simulink model "simumdl"  (Simulink 7.6)
settings: Solver=ode45  StartTime=0.0  StopTime=Tend  RelTol=1e-3
values from neighbouring files (symbols this model uses):
  A = 1    [contsid_MISO.m]
  B = [10 30]    [contsid_Hammerstein1.m]    (also in contsid_MISO.m = cell(1,2); B{1} = B1; B{2} = B2; contsid_RIVC.m = [2]; contsid_tutorial4.m = [-6400 1600]; contsid_tutorial5.m = K*wn^2*num)
  C = [1]    [contsid_Hammerstein1.m]    (also in contsid_HammersteinWiener1.m = sys0_ss.C; contsid_RIVC.m = [1 0.9])
  D = [1]    [contsid_Hammerstein1.m]    (also in contsid_HammersteinWiener1.m = sys0_ss.D; contsid_RIVC.m = [1 -1 .2])
  Dc = [1 0]    [contsid_closedloop1.m]
undefined symbols (not defined in the file or in its folder): Ac, Bc, Cc, Tsd
settings Model: Creator=pakjit  LastModifiedBy=pakjit
settings DataIOCC: LimitDataPoints=off  TimeSaveName=toutsim  OutputSaveName=youtsim

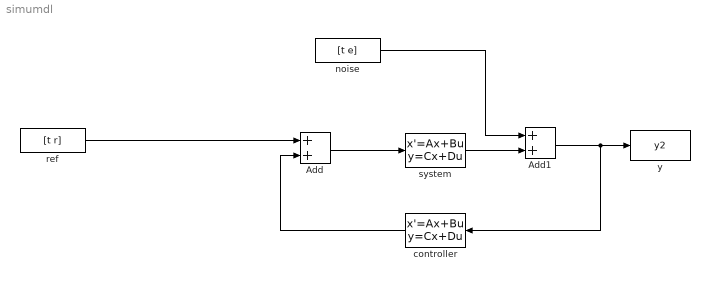
== system simumdl ==
  Add : Sum
  Add1 : Sum
  controller : StateSpace  A=Ac  B=Bc  C=Cc  D=Dc
  noise : FromWorkspace  VariableName=[t e]  SampleTime=0
  ref : FromWorkspace  VariableName=[t r]  SampleTime=0
  system : StateSpace  A=A  B=B  C=C  D=D
  y : ToWorkspace  VariableName=y2  SampleTime=Tsd  SaveFormat=Array
  wires:
  Add/1 -> system/1
  ref/1 -> Add/1
  noise/1 -> Add1/1
  system/1 -> Add1/2
  Add1/1 -> y/1, controller/1
  controller/1 -> Add/2
